simulink model "mpc_comp1"  (R2018a)
settings: Solver=ode45  StartTime=0.0  StopTime=8  RelTol=1e-3
values from neighbouring files (symbols this model uses):
  refs = [1;1]    [controlofnonlinearsystem.m]
libraries: cstblocks x1, mpclib x1
settings Model: ExtModeTrigMode=oneshot  ExtModeArmWhenConnect=off  Creator=The MathWorks, Inc.  LastModifiedBy=Nakul
settings DataIOCC: SaveFormat=Array  SignalLoggingName=sigsOut
settings OptimizationCC: BooleanDataType=off  ExpressionDepthLimit=2147483647  InitFltsAndDblsToZero=on  LifeSpan=inf
settings DebuggingCC: UnderspecifiedInitializationDetection=Classic  MergeDetectMultiDrivingBlocksExec=none  CheckExecutionContextPreStartOutputMsg=on  CheckExecutionContextRuntimeOutputMsg=on  SignalResolutionControl=TryResolveAllWithWarning  MultiTaskDSMMsg=warning  MultiTaskCondExecSysMsg=none  IntegerOverflowMsg=none  FcnCallInpInsideContextMsg=warning  StateNameClashWarn=warning  SFUnexpectedBacktrackingDiag=warning  SFNoUnconditionalDefaultTransitionDiag=warning  SFExecutionAtInitializationDiag=none  IntegerSaturationMsg=none
settings HardwareCC: ProdBitPerPointer=32  ProdBitPerSizeT=32  ProdBitPerPtrDiffT=32  ProdLargestAtomicFloat=None  ProdIntDivRoundTo=Undefined  ProdEndianess=Unspecified  ProdWordSize=32  ProdHWDeviceType=32-bit Generic  TargetUnknown=on
settings ModelReferenceCC: PropagateSignalLabelsOutOfModel=off
settings CodeAppCC: StateflowObjectComments=on
settings GRTTargetCC: TargetLangStandard=C89/C90 (ANSI)  GeneratePreprocessorConditionals=Disable all  CombineOutputUpdateFcns=off  GRTInterface=on
settings ConfigComp: CovMetricSettings=dw  CovHtmlReporting=on  CovSaveCumulativeToWorkspaceVar=on  CovSaveSingleToWorkspaceVar=on  CovExternalEMLEnable=off  CovSFcnEnable=off

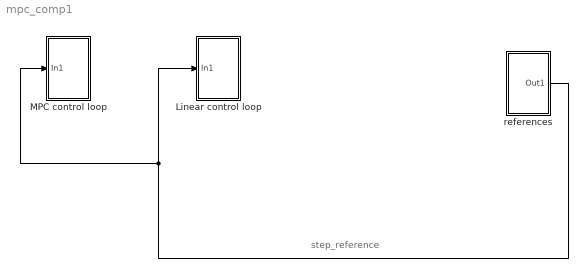
== system mpc_comp1 ==
  note: step_reference
  Linear control loop : Subsystem
  MPC control loop : Subsystem
  references : Subsystem
  wires:
  references/1(Out1) -> MPC control loop/1(In1), Linear control loop/1(In1)

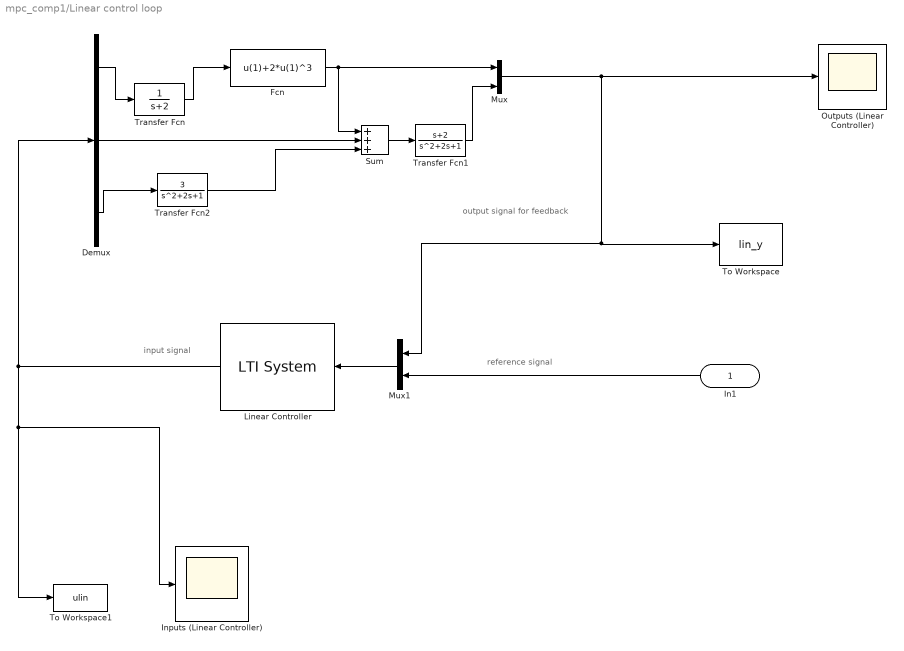
== system mpc_comp1/Linear control loop ==
  note: reference signal
  note: output signal
      | for feedback
  note: input signal
  In1 : Inport
  Demux : Demux  Outputs=3
  Fcn : Fcn  Expr=u(1)+2*u(1)^3
  Inputs (Linear Controller) : Scope
  Linear Controller : cstblocks/LTI System  sys=linear_contrllr  IC=0
  Mux : Mux  Inputs=2
  Mux1 : Mux  Inputs=2
  Outputs (Linear Controller) : Scope
  Sum : Sum  Inputs=+++  SaturateOnIntegerOverflow=on  InputSameDT=on  OutDataTypeStr=Inherit: Same as first input
  To Workspace : ToWorkspace  VariableName=lin_y  SampleTime=-1
      settings: MaxDataPoints=Inf
  To Workspace1 : ToWorkspace  VariableName=ulin  SampleTime=-1
      settings: MaxDataPoints=Inf
  Transfer Fcn : TransferFcn  Denominator=[1 2]
  Transfer Fcn1 : TransferFcn  Numerator=[1 2]
  Transfer Fcn2 : TransferFcn  Numerator=[3]
  wires:
  In1/1 -> Mux1/2
  Transfer Fcn1/1 -> Mux/2
  Demux/1 -> Transfer Fcn/1
  Sum/1 -> Transfer Fcn1/1
  Demux/2 -> Sum/2
  Fcn/1 -> Sum/1, Mux/1
  Transfer Fcn/1 -> Fcn/1
  Transfer Fcn2/1 -> Sum/3
  Demux/3 -> Transfer Fcn2/1
  Mux/1 -> Mux1/1, To Workspace/1, Outputs (Linear Controller)/1
  Linear Controller/1 -> Inputs (Linear Controller)/1, To Workspace1/1, Demux/1
  Mux1/1 -> Linear Controller/1

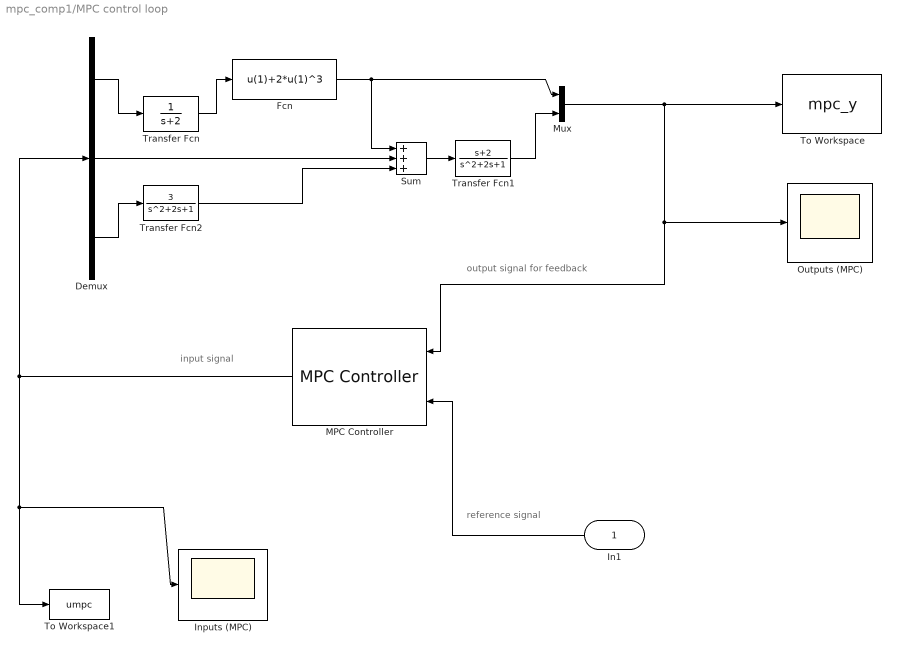
== system mpc_comp1/MPC control loop ==
  note: input signal
  note: output signal for feedback
  note: reference signal
  In1 : Inport
  Demux : Demux  Outputs=3
  Fcn : Fcn  Expr=u(1)+2*u(1)^3
  Inputs (MPC) : Scope
  MPC Controller : mpclib/MPC Controller  mpcobj=object1_mpc  x0=[]  is_multiple=0  enable_value=0  return_u0=off  updateMPCinCallerWorkspace=on  ref_from_ws=off  ref_signal_name=[]  ref_preview=on  md_from_ws=off  md_signal_name=[]  md_preview=on  from_project=off  project_file=MPCtask.mat  md_inport=off  mv_inport=off  cost_outport=off  return_sequence=off  return_qpstatus=off  return_state=off  state_inport=off  lims_inport=off  cc_inport=off  ywt_inport=off  is_designfromscratch=0  uwt_inport=off  duwt_inport=off  rhoeps_inport=off  uref_inport=off  n_ts=0.1  n_p=15  n_mv=3  n_md=0  n_ud=0  n_mo=2  n_uo=0  BlockDataType=double  SampleTimeInherited=off  switch_inport=off
  Mux : Mux  Inputs=2
  Outputs (MPC) : Scope
  Sum : Sum  Inputs=+++  SaturateOnIntegerOverflow=on  InputSameDT=on  OutDataTypeStr=Inherit: Same as first input
  To Workspace : ToWorkspace  VariableName=mpc_y  SampleTime=-1
      settings: MaxDataPoints=Inf
  To Workspace1 : ToWorkspace  VariableName=umpc  SampleTime=-1
      settings: MaxDataPoints=Inf
  Transfer Fcn : TransferFcn  Denominator=[1 2]
  Transfer Fcn1 : TransferFcn  Numerator=[1 2]
  Transfer Fcn2 : TransferFcn  Numerator=[3]
  wires:
  MPC Controller/1 -> Demux/1, Inputs (MPC)/1, To Workspace1/1
  Mux/1 -> MPC Controller/1, Outputs (MPC)/1, To Workspace/1
  Demux/3 -> Transfer Fcn2/1
  Transfer Fcn2/1 -> Sum/3
  Transfer Fcn/1 -> Fcn/1
  Fcn/1 -> Sum/1, Mux/1
  Demux/2 -> Sum/2
  Sum/1 -> Transfer Fcn1/1
  Demux/1 -> Transfer Fcn/1
  Transfer Fcn1/1 -> Mux/2
  In1/1 -> MPC Controller/2

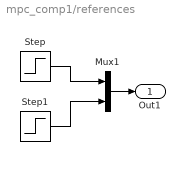
== system mpc_comp1/references ==
  Mux1 : Mux  Inputs=2
  Step : Step  Time=4  Before=refs(1)  After=0  SampleTime=0
  Step1 : Step  Time=0  After=refs(2)  SampleTime=0
  Out1 : Outport
  wires:
  Step/1 -> Mux1/1
  Step1/1 -> Mux1/2
  Mux1/1 -> Out1/1
